simulink model "probe_FSM"  (R2020a)
settings: Solver=FixedStepAuto  StartTime=0.0  StopTime=10.0  RelTol=1e-3
libraries: androiduilib x9
settings Model: Creator=sebastian  LastModifiedBy=corte
settings OptimizationCC: EnhancedBackFolding=on  PassReuseOutputArgsAs=Individual arguments  ZeroExternalMemoryAtStartup=off  ZeroInternalMemoryAtStartup=off  MaxStackSize=64  OptimizeBlockOrder=speed  DifferentSizesBufferReuse=on  OptimizationCustomize=off  EfficientTunableParamExpr=on
settings DebuggingCC: ParameterTunabilityLossMsg=error
settings HardwareCC: ProdBitPerPointer=32  ProdBitPerSizeT=32  ProdBitPerPtrDiffT=32  ProdLargestAtomicInteger=Long  ProdLargestAtomicFloat=Double  ProdWordSize=32  ProdHWDeviceType=ARM Compatible->ARM Cortex
settings SFSimCC: MATLABDynamicMemAlloc=off
settings RTWCC: SystemTargetFile=ert.tlc  HardwareBoard=Android Device  TemplateMakefile=ert_default_tmf  RTWVerbose=off  Toolchain=Android SDK/NDK Tools
settings CodeAppCC: ForceParamTrailComments=on  IgnoreCustomStorageClasses=off  OperatorAnnotations=on  SimulinkDataObjDesc=on  SFDataObjDesc=on  InsertBlockDesc=on

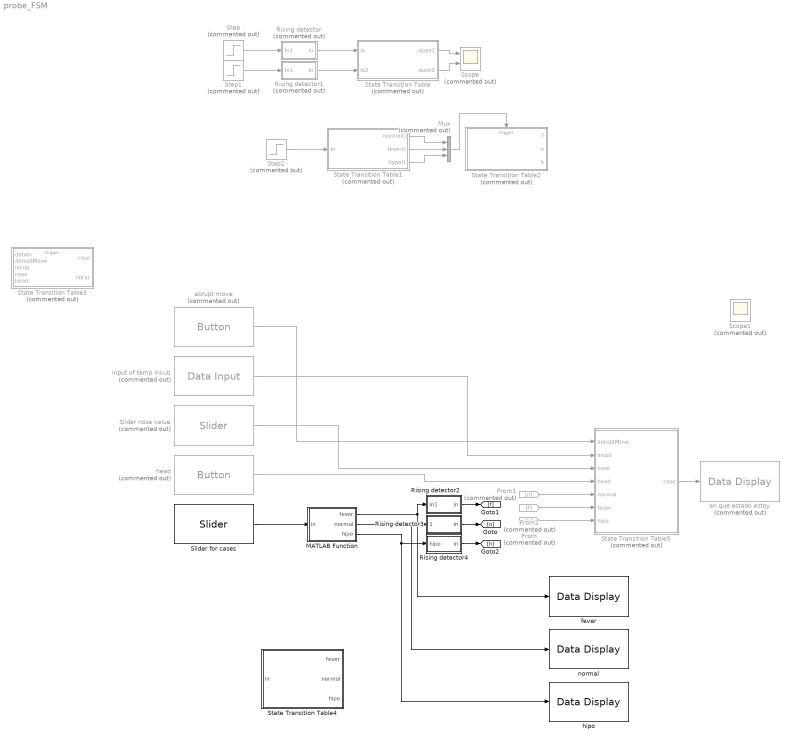
== system probe_FSM ==
  From : From  Commented=on  GotoTag=h
  From1 : From  Commented=on  GotoTag=n
  From2 : From  Commented=on  GotoTag=f
  MATLAB Function : MATLAB Function  TreatAsAtomicUnit=on
  Mux : Mux  Commented=on  Inputs=3
  Rising detector : Subsystem  Commented=on
  Rising detector1 : Subsystem  Commented=on
  Rising detector2 : Subsystem
  Rising detector3 : Subsystem
  Rising detector4 : Subsystem
  Scope : Scope  Commented=on  NumInputPorts=2
  Scope1 : Scope  Commented=on
  Slider for cases : androiduilib/Slider  Min=0  Value=0  Max=3  Resolution=1  SliderId=probe_FSM/Slider_for_cases  SampleTime=0.1  BlockPlatform=Android
      settings: SourceProductBaseCode=ANDROID
  Slider nose value : androiduilib/Slider  Commented=on  Min=0  Value=0  Max=3  Resolution=1  SliderId=probe_FSM/Slider_nose_value  SampleTime=0.1  BlockPlatform=Android
      settings: SourceProductBaseCode=ANDROID
  State Transition Table : State Transition Table  Commented=on  TreatAsAtomicUnit=on
  State Transition Table1 : State Transition Table  Commented=on  TreatAsAtomicUnit=on
  State Transition Table2 : State Transition Table  Commented=on  TreatAsAtomicUnit=on
  State Transition Table3 : State Transition Table  Commented=on  TreatAsAtomicUnit=on
  State Transition Table4 : State Transition Table  TreatAsAtomicUnit=on
  State Transition Table5 : State Transition Table  Commented=on  TreatAsAtomicUnit=on
  Step : Step  Commented=on  SampleTime=0
  Step1 : Step  Commented=on  Time=2  SampleTime=0
  Step2 : Step  Commented=on  After=2  SampleTime=0
  abrupt move : androiduilib/Button  Commented=on  ButtonState=Not pressed  ButtonId=probe_FSM/abrupt_move  State=off  SampleTime=0.1  BlockPlatform=Android
      settings: SourceProductBaseCode=ANDROID
  en que estado estoy : androiduilib/Data Display  Commented=on  DataDisplayId=probe_FSM/en_que_estado_estoy  Format=Float  Precision=6  SimulateUsing=Code generation  blockPlatform=Android
      settings: SourceProductBaseCode=ANDROID
  fever : androiduilib/Data Display  DataDisplayId=probe_FSM/fever  Format=Float  Precision=6  SimulateUsing=Code generation  blockPlatform=Android
      settings: SourceProductBaseCode=ANDROID
  head : androiduilib/Button  Commented=on  ButtonState=Not pressed  ButtonId=probe_FSM/head  State=off  SampleTime=0.1  BlockPlatform=Android
      settings: SourceProductBaseCode=ANDROID
  hipo : androiduilib/Data Display  DataDisplayId=probe_FSM/hipo  Format=Float  Precision=6  SimulateUsing=Code generation  blockPlatform=Android
      settings: SourceProductBaseCode=ANDROID
  input of temp incub : androiduilib/Data Input  Commented=on  isCharVector=off  Value=26  CharVector=Hello World  OutputDataType=double  maxCharVectorSize=100  DataInputId=probe_FSM/input_of_temp_incub  SampleTime=0.1
      settings: SourceProductBaseCode=ANDROID
  normal : androiduilib/Data Display  DataDisplayId=probe_FSM/normal  Format=Float  Precision=6  SimulateUsing=Code generation  blockPlatform=Android
      settings: SourceProductBaseCode=ANDROID
  wires:
  Rising detector/1(in) -> State Transition Table/1(in)
  Step/1 -> Rising detector/1(In1)
  Rising detector1/1(in) -> State Transition Table/2(in2)
  Step1/1 -> Rising detector1/1(In1)
  State Transition Table/1(state1) -> Scope/1
  State Transition Table/2(state2) -> Scope/2
  Step2/1 -> State Transition Table1/1(in)
  Mux/1 -> State Transition Table2/Trigger
  State Transition Table1/1(normal()) -> Mux/1
  State Transition Table1/2(fever()) -> Mux/2
  State Transition Table1/3(hypo()) -> Mux/3
  Rising detector3/1(in) -> [n]
  Rising detector2/1(in) -> [f]
  Rising detector4/1(in) -> [h]
  From2/1 -> State Transition Table5/6(fever)
  From/1 -> State Transition Table5/7(hipo)
  From1/1 -> State Transition Table5/5(normal)
  Slider for cases/1 -> MATLAB Function/1(in)
  MATLAB Function/1(fever) -> Rising detector2/1(In1), fever/1
  MATLAB Function/2(normal) -> normal/1, Rising detector3/1(normal)
  MATLAB Function/3(hipo) -> hipo/1, Rising detector4/1(hipo)
  input of temp incub/1 -> State Transition Table5/2(incub)
  abrupt move/1 -> State Transition Table5/1(abruptMove)
  Slider nose value/1 -> State Transition Table5/3(nose)
  head/1 -> State Transition Table5/4(head)
  State Transition Table5/1(caso) -> en que estado estoy/1

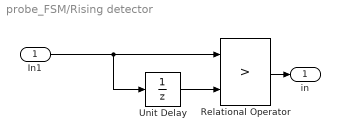
== system probe_FSM/Rising detector ==
  In1 : Inport
  Relational Operator : RelationalOperator  Operator=>  OutDataTypeStr=boolean  RndMeth=Simplest
  Unit Delay : UnitDelay  SampleTime=-1  HasFrameUpgradeWarning=on
  in : Outport
  wires:
  Unit Delay/1 -> Relational Operator/2
  In1/1 -> Unit Delay/1, Relational Operator/1
  Relational Operator/1 -> in/1

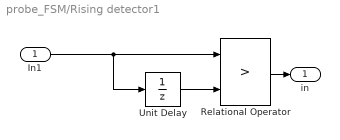
== system probe_FSM/Rising detector1 ==
  In1 : Inport
  Relational Operator : RelationalOperator  Operator=>  OutDataTypeStr=boolean  RndMeth=Simplest
  Unit Delay : UnitDelay  SampleTime=-1  HasFrameUpgradeWarning=on
  in : Outport
  wires:
  Relational Operator/1 -> in/1
  In1/1 -> Relational Operator/1, Unit Delay/1
  Unit Delay/1 -> Relational Operator/2

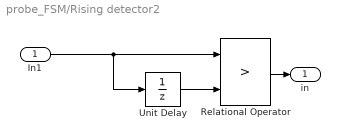
== system probe_FSM/Rising detector2 ==
  In1 : Inport
  Relational Operator : RelationalOperator  Operator=>  OutDataTypeStr=boolean  RndMeth=Simplest
  Unit Delay : UnitDelay  SampleTime=-1  HasFrameUpgradeWarning=on
  in : Outport
  wires:
  Unit Delay/1 -> Relational Operator/2
  In1/1 -> Unit Delay/1, Relational Operator/1
  Relational Operator/1 -> in/1

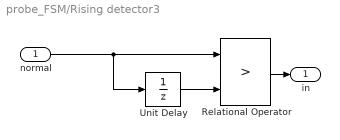
== system probe_FSM/Rising detector3 ==
  normal : Inport
  Relational Operator : RelationalOperator  Operator=>  OutDataTypeStr=boolean  RndMeth=Simplest
  Unit Delay : UnitDelay  SampleTime=-1  HasFrameUpgradeWarning=on
  in : Outport
  wires:
  Relational Operator/1 -> in/1
  normal/1 -> Relational Operator/1, Unit Delay/1
  Unit Delay/1 -> Relational Operator/2

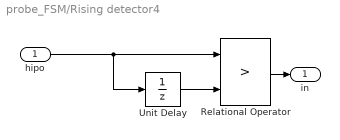
== system probe_FSM/Rising detector4 ==
  hipo : Inport
  Relational Operator : RelationalOperator  Operator=>  OutDataTypeStr=boolean  RndMeth=Simplest
  Unit Delay : UnitDelay  SampleTime=-1  HasFrameUpgradeWarning=on
  in : Outport
  wires:
  Unit Delay/1 -> Relational Operator/2
  hipo/1 -> Unit Delay/1, Relational Operator/1
  Relational Operator/1 -> in/1

== stateflow chart probe_FSM/State Transition Table1 ==
  state init
  state case_normal
  state case_fever
  state case_hipo
  (default) -> init
  (junction 36) -> init
  (junction 38) -> (junction 36)
  init -> case_normal : after(1,sec)
  case_normal -> (junction 41) [order 1] : [in == 0]
      | {normal}
  (junction 41) -> case_normal
  case_normal -> case_fever [order 2]
  case_fever -> (junction 29) [order 1] : [in == 1]
      | {fever}
  (junction 29) -> case_fever
  case_fever -> case_hipo [order 2]
  case_hipo -> (junction 33) [order 1] : [in == 2]
      | {hypo}
  (junction 33) -> case_hipo
  case_hipo -> (junction 38) [order 2]
  data: in input
  events: normal output FUNCTION_CALL_EVENT; fever output FUNCTION_CALL_EVENT; hypo output FUNCTION_CALL_EVENT

== stateflow chart probe_FSM/State Transition Table2 ==
  state init
  state normal
    f = 0;
    n = 1;
    h = 0;
  state fever
    f = 1;
    n = 0;
    h = 0;
  state hipo
    h = 1;
    f = 0;
    n = 0;
  (default) -> init
  (junction 36) -> init
  init -> (junction 23) [order 2] : [fever()]
  (junction 38) -> (junction 36)
  (junction 23) -> (junction 21)
  init -> (junction 32) [order 3] : [hypo()]
  (junction 32) -> (junction 30)
  init -> normal [order 1] : [normal()]
  normal -> init
  fever -> (junction 38)
  (junction 21) -> fever
  (junction 41) -> (junction 38)
  hipo -> (junction 41)
  (junction 30) -> hipo
  data: f output; n output; h output
  events: normal input FUNCTION_CALL_EVENT; fever input FUNCTION_CALL_EVENT; hypo input FUNCTION_CALL_EVENT

== stateflow chart probe_FSM/State Transition Table3 ==
  state saludable
    caso=0;
    llorar = 0;
  state fiebre
    caso = 1;
    llorar = 1;
  state hipotermia
    caso = -2;
    llorar = 1;
  state agitado
    caso = 3.5;
    llorar = 1;
  (default) -> saludable
  (junction 40) -> saludable
  (junction 42) -> (junction 40)
  saludable -> (junction 28) [order 2] : [datain == 2]
  (junction 28) -> (junction 26)
  saludable -> fiebre [order 1] : [fever()]
  fiebre -> saludable [order 1] : [normal()]
  fiebre -> saludable [order 3] : [incub > 23 && incub <= 25 && nose == 2]
      | {}
  saludable -> (junction 73) [order 3] : [abruptMove == 1]
  (junction 73) -> (junction 31)
  (junction 60) -> fiebre
  (junction 62) -> (junction 60)
  fiebre -> hipotermia [order 2] : [datain == 2]
  fiebre -> hipotermia [order 4] : [incub < 23]
  hipotermia -> fiebre [order 2] : [fever()]
  hipotermia -> fiebre [order 4] : [incub > 30]
  hipotermia -> (junction 42) [order 1] : [normal()]
  (junction 103) -> (junction 42)
  hipotermia -> (junction 103) [order 3] : [incub > 29 && incub <= 30 && head == 1]
  (junction 137) -> (junction 103)
  (junction 26) -> hipotermia
  agitado -> hipotermia [order 3] : [datain == 2]
  agitado -> (junction 62) [order 2] : [fever]
  agitado -> (junction 137) [order 1] : [normal()]
  (junction 31) -> agitado
  data: datain input; caso output; abruptMove input; llorar output; incub input; nose input; head input
  events: normal input FUNCTION_CALL_EVENT; fever input FUNCTION_CALL_EVENT; hypo input FUNCTION_CALL_EVENT

== stateflow chart probe_FSM/State Transition Table ==
  state estado_1
    state1=1;
    state2=0;
  state estado_2
    state2=1;
    state1=0;
  (default) -> estado_1
  estado_1 -> estado_2 : [in]
  estado_2 -> estado_1 : [in2]
  data: in input; in2 input; state1 output; state2 output

== stateflow chart probe_FSM/State Transition Table4 ==
  state init
  state case_normal
    normal = 1;
    fever = 0;
    hipo = 0;
  state case_fever
    normal = 0;
    fever = 1;
    hipo = 0;
  state case_hipo
    normal = 0;
    fever = 0;
    hipo = 1;
  (default) -> init
  (junction 36) -> init
  init -> (junction 49) [order 2] : [in == 1]
  (junction 58) -> (junction 36)
  (junction 49) -> (junction 47)
  init -> (junction 54) [order 3] : [in == 2]
  (junction 54) -> (junction 52)
  init -> case_normal [order 1] : [in == 0]
  case_normal -> init : after(0.1,sec)
  case_fever -> (junction 58) : after(0.1,sec)
  (junction 61) -> (junction 58)
  (junction 47) -> case_fever
  case_hipo -> (junction 61) : after(0.1,sec)
  (junction 52) -> case_hipo
  data: in input; fever output; normal output; hipo output

== stateflow chart probe_FSM/State Transition Table5 ==
  state saludable
    caso=0;
  state fiebre
    caso = 1;
  state hipotermia
    caso = 2;
  state agitado
    caso = 3;
  (default) -> saludable
  (junction 40) -> saludable
  (junction 42) -> (junction 40)
  saludable -> (junction 28) [order 2] : [hipo == 1]
  (junction 28) -> (junction 26)
  saludable -> fiebre [order 1] : [fever == 1]
  fiebre -> saludable [order 1] : [normal == 1]
  fiebre -> saludable [order 3] : [incub > 23 && incub <= 25 && nose == 2]
      | {}
  saludable -> (junction 73) [order 3] : [abruptMove == 1]
  (junction 73) -> (junction 31)
  (junction 60) -> fiebre
  (junction 62) -> (junction 60)
  fiebre -> hipotermia [order 2] : [hipo == 1]
  fiebre -> hipotermia [order 4] : [incub < 23]
  hipotermia -> fiebre [order 2] : [fever == 1]
  hipotermia -> fiebre [order 4] : [incub > 30]
  hipotermia -> (junction 42) [order 1] : [normal == 1]
  (junction 103) -> (junction 42)
  hipotermia -> (junction 103) [order 3] : [incub > 29 && incub <= 30 && head == 1]
  (junction 45) -> (junction 103)
  (junction 26) -> hipotermia
  agitado -> hipotermia [order 3] : [hipo == 1]
  agitado -> (junction 45) [order 1] : [normal == 1]
  (junction 136) -> (junction 45)
  agitado -> (junction 62) [order 2] : [fever == 1]
  agitado -> (junction 136) [order 4] : after(5,sec)
  (junction 31) -> agitado
  data: caso output; abruptMove input; incub input; nose input; head input; normal input; fever input; hipo input

== matlab function probe_FSM/MATLAB Function ==
  data: in input; fever output; normal output; hipo output
function [fever, normal, hipo] = fcn(in)

if in == 0
    normal = 1; 
    fever = 0; 
    hipo = 0;
elseif in == 1
    normal = 0; 
    fever = 1; 
    hipo = 0; 
elseif in == 2
    normal = 0; 
    fever = 0; 
    hipo = 1;
else
    normal = 0; 
    fever = 0; 
    hipo = 0;
end
